simulink model "bh_3d_pend_LINEARIZE_harness"  (R2017a)
settings: Solver=ode45  StartTime=0.0  StopTime=11  RelTol=1e-5  EnableMultiTasking=on
settings Model: Creator=bhorton  LastModifiedBy=bhorton
settings SolverCC: ZeroCrossAlgorithm=Adaptive
settings DataIOCC: LimitDataPoints=on
settings OptimizationCC: LifeSpan=inf
settings DebuggingCC: AllowSymbolicDim=off  SFUnexpectedBacktrackingDiag=warning  SFNoUnconditionalDefaultTransitionDiag=warning  SFExecutionAtInitializationDiag=none
settings GRTTargetCC: TargetLangStandard=C89/C90 (ANSI)  GeneratePreprocessorConditionals=Disable all
settings ConfigComp: CovMetricSettings=dw  CovHtmlReporting=on  CovSaveCumulativeToWorkspaceVar=on  CovSaveSingleToWorkspaceVar=on  CovExternalEMLEnable=off  CovSFcnEnable=off
settings SimscapeCC: SimscapeLogType=all  SimscapeLogDataHistory=10000
settings ConfigurationSet: Description=SimMechanics 2G

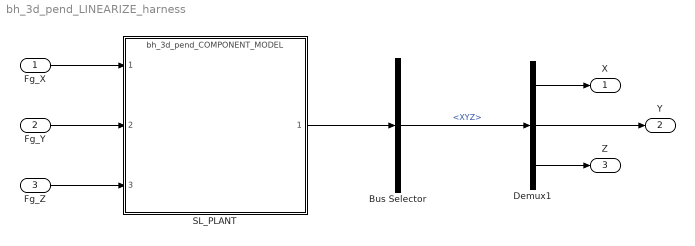
== system bh_3d_pend_LINEARIZE_harness ==
  Fg_X : Inport
  Fg_Y : Inport  Port=2
  Fg_Z : Inport  Port=3
  Bus Selector : BusSelector  OutputSignals=XYZ
  Demux1 : Demux  Outputs=3
  SL_PLANT : ModelReference  ModelNameDialog=bh_3d_pend_COMPONENT_MODEL.slx  SimulationMode=Normal  ModelReferenceVersion=1.14
  X : Outport
  Y : Outport  Port=2
  Z : Outport  Port=3
  wires:
  Fg_Z/1 -> SL_PLANT/3
  Fg_Y/1 -> SL_PLANT/2
  Fg_X/1 -> SL_PLANT/1
  SL_PLANT/1 -> Bus Selector/1
  Bus Selector/1 -> Demux1/1  "<XYZ>"
  Demux1/2 -> Y/1
  Demux1/1 -> X/1
  Demux1/3 -> Z/1
